simulink model "Ld_Lq_realised_inverter_sinPWM"  (R2021b)
settings: Solver=ode23tb  StartTime=0.0  StopTime=0.16  MaxStep=5e-6  RelTol=1e-3  EnableMultiTasking=on
libraries: spsSeriesRLCBranchLib x18, spsCurrentMeasurementLib x8, spsVoltageMeasurementLib x8, spsMosfetLib x6, simulink x3, spsIdealSwitchLib x1, slpidlib x1, spsThreePhaseSourceLib x1, spspowerguiLib x1
settings Model: SimulationMode=accelerator  Creator=Алексей  LastModifiedBy=alexey
settings SolverCC: ZeroCrossControl=DisableAll  ZeroCrossAlgorithm=Adaptive  AlgebraicLoopSolver=TrustRegion
settings DataIOCC: SaveFormat=Array  SaveOutput=off  SignalLogging=off  DSMLogging=off  SaveTime=off  ReturnWorkspaceOutputs=off
settings OptimizationCC: LifeSpan=inf
settings DebuggingCC: UnderspecifiedInitializationDetection=Classic  MergeDetectMultiDrivingBlocksExec=none  SolverPrmCheckMsg=warning  AllowSymbolicDim=off  SFUnexpectedBacktrackingDiag=warning  SFNoUnconditionalDefaultTransitionDiag=warning  SFExecutionAtInitializationDiag=none  SFMachineParentedDataDiag=warning  ArithmeticOperatorsInVariantConditions=warning
settings HardwareCC: ProdBitPerPointer=32  ProdBitPerSizeT=32  ProdBitPerPtrDiffT=32  ProdLargestAtomicFloat=None  ProdIntDivRoundTo=Undefined  ProdEndianess=Unspecified  ProdWordSize=32  ProdHWDeviceType=32-bit Generic
settings ModelReferenceCC: PropagateSignalLabelsOutOfModel=off
settings SFSimCC: SimUseLocalCustomCode=off  CustomCodeUndefinedFunction=UseInterfaceOnly
settings RTWCC: RTWUseLocalCustomCode=off
settings CodeAppCC: StateflowObjectComments=on
settings GRTTargetCC: TargetLangStandard=C89/C90 (ANSI)  RTWCAPISignals=on  RTWCAPIParams=on
settings ConfigComp: CovMetricSettings=dw  CovSaveCumulativeToWorkspaceVar=on  CovSaveSingleToWorkspaceVar=on  CovExternalEMLEnable=off  CovSFcnEnable=off
settings SimscapeCC: SimscapeNormalizeSystem=off

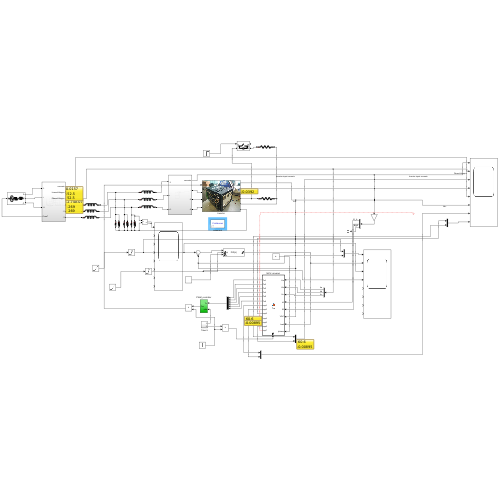
[thumbnail: Simulink's stored preview of the top-level diagram]
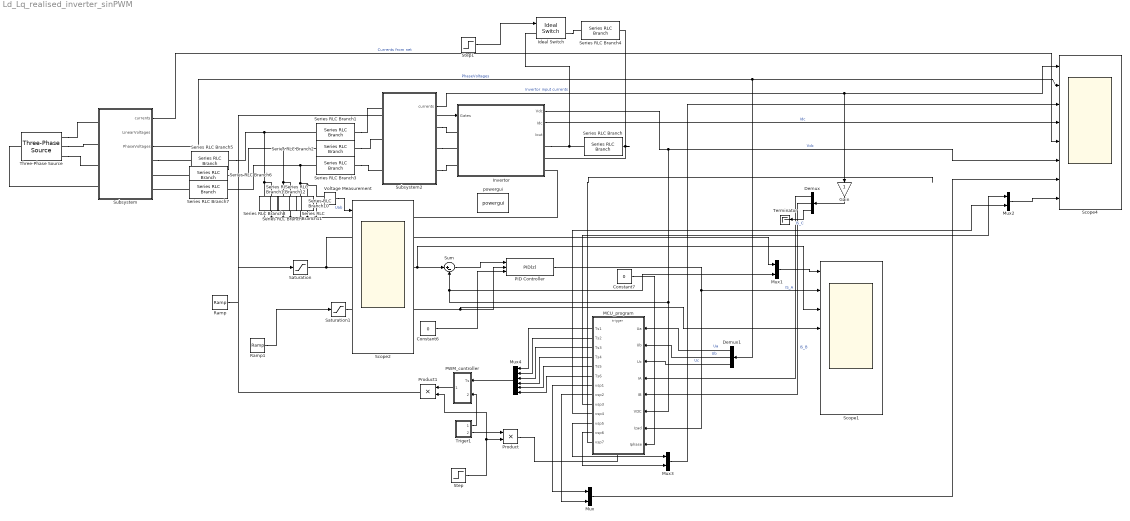
== system Ld_Lq_realised_inverter_sinPWM ==
  Constant6 : Constant  Value=0
  Constant7 : Constant  Value=0
  Demux : Demux  Outputs=3
  Demux1 : Demux  Outputs=3
  Gain : Gain
  Ideal Switch : spsIdealSwitchLib/Ideal Switch  Ron=0.001  Lon=0  IC=0  Rs=1e5  Cs=inf  Measurements=on
  Invertor : Subsystem
      mask Display: image('$imagefile'); % Use "Edit Image" on toolstrip to change.
  MCU_program : MATLAB Function  TreatAsAtomicUnit=on
  Mux{,1..3} (4 alike) : Mux  Inputs=2
  Mux4 : Mux  Inputs=6
  PID Controller : slpidlib/PID Controller  Controller=PID  Form=Parallel  TimeDomain=Discrete-time  UseExternalTs=off  SampleTime=50e-6  IntegratorMethod=Forward Euler  FilterMethod=Forward Euler  ControllerParametersSource=internal  P=3  I=15  D=0  UseFilter=on  N=100  TunerSelectOption=Transfer Function Based (PID Tuner App)  InitialConditionSource=internal  InitialConditionForIntegrator=0  InitialConditionForFilter=0  DifferentiatorICPrevScaledInput=0  ExternalReset=none  TrackingMode=off  Kt=1  LimitOutput=on  SatLimitsSource=external  UpperSaturationLimit=150  LowerSaturationLimit=0  LinearizeAsGain=on  AntiWindupMode=clamping  Kb=1  POutMin=[]  POutMax=[]  IOutMin=[]  IOutMax=[]  DOutMin=[]  DOutMax=[]  NOutMin=[]  NOutMax=[]  SumOutMin=[]  SumOutMax=[]  SaturationOutMin=[]  SaturationOutMax=[]  PParamMin=[]  PParamMax=[]  IParamMin=[]  IParamMax=[]  DParamMin=[]  DParamMax=[]  NParamMin=[]  NParamMax=[]  KbParamMin=[]  KbParamMax=[]  KtParamMin=[]  KtParamMax=[]  KbOutMin=[]  KbOutMax=[]  KtOutMin=[]  KtOutMax=[]  IntegratorOutMin=[]  IntegratorOutMax=[]  FilterOutMin=[]  FilterOutMax=[]  SumI1OutMin=[]  SumI1OutMax=[]  SumI2OutMin=[]  SumI2OutMax=[]  SumI3OutMin=[]  SumI3OutMax=[]  SumI4OutMin=[]  SumI4OutMax=[]  SumDOutMin=[]  SumDOutMax=[]  DifferentiatorOutMin=[]  DifferentiatorOutMax=[]  FilterDiffOutCoefMin=[]  FilterDiffOutCoefMax=[]  ReciprocalOutMin=[]  ReciprocalOutMax=[]  SumDenOutMin=[]  SumDenOutMax=[]  SumNumOutMin=[]  SumNumOutMax=[]  DivideOutMin=[]  DivideOutMax=[]  UdiffTsProdOutMin=[]  UdiffTsProdOutMax=[]  NTsProdOutMin=[]  NTsProdOutMax=[]  UintegralTsProdOutMin=[]  UintegralTsProdOutMax=[]  UngainTsProdOutMin=[]  UngainTsProdOutMax=[]  IntegratorContinuousStateAttributes=''  IntegratorStateMustResolveToSignalObject=off  IntegratorRTWStateStorageClass=Auto  FilterContinuousStateAttributes=''  FilterStateMustResolveToSignalObject=off  FilterRTWStateStorageClass=Auto  ParallelPVariant=InternalParameters  IdealPVariant=Disabled  IVariant=InternalParameters  DVariant=InternalParameters  IntegratorVariant=Discrete  SatVariant=External  AWVariant=DiscClampingParallel  PCopyVariant=Disabled  TRVariant=Disabled  FdbkBlocksVariant=Forward  IdealPFdbkVariant=Disabled  SatFdbkVariant=Disabled  DerivativeFilterVariant=ForwardEulerFilter  NVariant=InternalParameters  NCopyVariant=Disabled  FilterICVariant=InternalICsFilter  IntegratorICVariant=InternalICs  ExternalResetVariant=Disabled  TRSumVariant=Passthrough  SumFdbkVariant=Disabled  SumVariant=Sum_PID  TsampFilterVariant=InternalTs  TsampNgainVariant=Passthrough  TsampIntegralVariant=Passthrough  ExternalSaturationOutDataTypeStr=Inherit: Same as second input
  PWM_controller : Subsystem
  Product : Product
  Product1 : Product
  Ramp : simulink/Sources/Ramp  slope=6500  start=0  InitialOutput=550
  Ramp1 : simulink/Sources/Ramp  slope=15000  start=0  InitialOutput=0
  Saturation : Saturate  UpperLimit=650  LowerLimit=560
  Saturation1 : Saturate  UpperLimit=150  LowerLimit=50
  Scope1 : Scope  NumInputPorts=8
  Scope2 : Scope  NumInputPorts=8
  Scope4 : Scope  NumInputPorts=8
  Series RLC Branch : spsSeriesRLCBranchLib/Series RLC Branch  LConnTagsString=__new0  RConnTagsString=__new0  BranchType=R  Resistance=50  Inductance=1e-3  SetiL0=off  InitialCurrent=0  Capacitance=1e-6  Setx0=off  InitialVoltage=0  Measurements=None
  Series RLC Branch1 : spsSeriesRLCBranchLib/Series RLC Branch  LConnTagsString=__new0  RConnTagsString=__new0  BranchType=L  Resistance=10  Inductance=500e-6  SetiL0=off  InitialCurrent=0  Capacitance=1e-6  Setx0=off  InitialVoltage=0  Measurements=None
  Series RLC Branch10 : spsSeriesRLCBranchLib/Series RLC Branch  LConnTagsString=__new0  RConnTagsString=__new0  BranchType=C  Resistance=10  Inductance=750e-6  SetiL0=off  InitialCurrent=0  Capacitance=1e-12  Setx0=off  InitialVoltage=0  Measurements=None
  Series RLC Branch11 : spsSeriesRLCBranchLib/Series RLC Branch  LConnTagsString=__new0  RConnTagsString=__new0  BranchType=R  Resistance=1e6  Inductance=750e-6  SetiL0=off  InitialCurrent=0  Capacitance=2e-18  Setx0=off  InitialVoltage=0  Measurements=None
  Series RLC Branch12 : spsSeriesRLCBranchLib/Series RLC Branch  LConnTagsString=__new0  RConnTagsString=__new0  BranchType=R  Resistance=1e6  Inductance=750e-6  SetiL0=off  InitialCurrent=0  Capacitance=2e-18  Setx0=off  InitialVoltage=0  Measurements=None
  Series RLC Branch13 : spsSeriesRLCBranchLib/Series RLC Branch  LConnTagsString=__new0  RConnTagsString=__new0  BranchType=R  Resistance=1e6  Inductance=750e-6  SetiL0=off  InitialCurrent=0  Capacitance=2e-18  Setx0=off  InitialVoltage=0  Measurements=None
  Series RLC Branch2 : spsSeriesRLCBranchLib/Series RLC Branch  LConnTagsString=__new0  RConnTagsString=__new0  BranchType=L  Resistance=10  Inductance=500e-6  SetiL0=off  InitialCurrent=0  Capacitance=1e-6  Setx0=off  InitialVoltage=0  Measurements=None
  Series RLC Branch3 : spsSeriesRLCBranchLib/Series RLC Branch  LConnTagsString=__new0  RConnTagsString=__new0  BranchType=L  Resistance=10  Inductance=500e-6  SetiL0=off  InitialCurrent=0  Capacitance=1e-6  Setx0=off  InitialVoltage=0  Measurements=None
  Series RLC Branch4 : spsSeriesRLCBranchLib/Series RLC Branch  LConnTagsString=__new0  RConnTagsString=__new0  BranchType=R  Resistance=20  Inductance=1e-3  SetiL0=off  InitialCurrent=0  Capacitance=1e-6  Setx0=off  InitialVoltage=0  Measurements=None
  Series RLC Branch5 : spsSeriesRLCBranchLib/Series RLC Branch  LConnTagsString=__new0  RConnTagsString=__new0  BranchType=L  Resistance=10  Inductance=5e-6  SetiL0=off  InitialCurrent=0  Capacitance=1e-6  Setx0=off  InitialVoltage=0  Measurements=None
  Series RLC Branch6 : spsSeriesRLCBranchLib/Series RLC Branch  LConnTagsString=__new0  RConnTagsString=__new0  BranchType=L  Resistance=10  Inductance=5e-6  SetiL0=off  InitialCurrent=0  Capacitance=1e-6  Setx0=off  InitialVoltage=0  Measurements=None
  Series RLC Branch7 : spsSeriesRLCBranchLib/Series RLC Branch  LConnTagsString=__new0  RConnTagsString=__new0  BranchType=L  Resistance=10  Inductance=5e-6  SetiL0=off  InitialCurrent=0  Capacitance=1e-6  Setx0=off  InitialVoltage=0  Measurements=None
  Series RLC Branch8 : spsSeriesRLCBranchLib/Series RLC Branch  LConnTagsString=__new0  RConnTagsString=__new0  BranchType=C  Resistance=10  Inductance=750e-6  SetiL0=off  InitialCurrent=0  Capacitance=1e-12  Setx0=off  InitialVoltage=0  Measurements=None
  Series RLC Branch9 : spsSeriesRLCBranchLib/Series RLC Branch  LConnTagsString=__new0  RConnTagsString=__new0  BranchType=C  Resistance=10  Inductance=750e-6  SetiL0=off  InitialCurrent=0  Capacitance=1e-12  Setx0=off  InitialVoltage=0  Measurements=None
  Step : Step  Time=0  SampleTime=0
  Step1 : Step  Time=0.1  SampleTime=0
  Subsystem : Subsystem
  Subsystem2 : Subsystem
  Sum : Sum  Inputs=|+-
  Terminator : Terminator
  Three-Phase Source : spsThreePhaseSourceLib/Three-Phase Source  InternalConnection=Yn  VoltagePhases=on  Voltage=200  PhaseAngle=0  Voltage_phases=[220 220 220]  PhaseAngles_phases=[0 -120 +120]  Frequency=50  NonIdealSource=on  SpecifyImpedance=off  Resistance=1e-6  Inductance=30e-9  ShortCircuitLevel=100e6  BaseVoltage=200  XRratio=7  BusType=swing  Pref=10e3  Qref=0  Prefabc=[10e3, 10e3, 10e3]  Qrefabc=[0, 0, 0]  Qmin=-inf  Qmax=inf
  Triger1 : Subsystem
  Voltage Measurement : spsVoltageMeasurementLib/Voltage Measurement  PhasorSimulation=off  OutputType=Complex  PSBequivalent=0
  powergui : spspowerguiLib/powergui  Priority=1  SimulationMode=Continuous  SampleTime=50e-6  frequency=60  Iterations=50  frequencyindice=0  Pbase=100e6  ErrMax=1e-4  UnitsV=kV  UnitsW=MW  buscounter=0  FunctionMessages=off  echomessages=off  EnableUseOfTLC=off  CurrentSourceSwitches=on  DisableSnubberDevices=off  DisableRonSwitches=off  DisableVfSwitches=off  DisplayEquations=off  AutomaticDiscreteSolvers=off  SolverType=Tustin  Interpol=off  ExternalGateDelay=off  methode=off  Ts=0  x0status=blocks  SPID=off  SwTol=0  HookPort=off  NonlinearTolerance=1e-4  nMaxIteration=100  ContinueOnMaxIteration=off  RestoreLinks=warning  ResistiveCurrentMeasurement=off  Frange=[0:2:500]  Ylog=off  Xlog=on  ShowGrid=off  save=off  variable=ZData  structure=SD2  ZoomFFT=on  StartTime=0.7  cycles=10  DisplayStyle=4  fundamental=382  FreqAxis=off  MaxFrequency=50000  frequencyindicesteady=1  RmsSteady=1  display=off
  wires:
  Demux/1 -> MCU_program/4(IA)  "IS_A"
  Demux/2 -> MCU_program/5(IB)  "IS_B"
  MCU_program/8(vsp2) -> Mux/2
  MCU_program/7(vsp1) -> Mux/1
  MCU_program/6(Ts6) -> Mux4/6
  MCU_program/5(Ts5) -> Mux4/5
  MCU_program/4(Ts4) -> Mux4/4
  MCU_program/3(Ts3) -> Mux4/3
  Triger1/1(1) -> PWM_controller/2(pila)
  Product1/1 -> Invertor/1(Gates)
  MCU_program/1(Ts1) -> Mux4/1
  Mux4/1 -> PWM_controller/1(Ts)
  Product/1 -> MCU_program/Trigger
  MCU_program/2(Ts2) -> Mux4/2
  Invertor/1(Vdc) -> Scope4/6, Mux1/2, Sum/2, MCU_program/6(VDC)  "Vdc"
  Invertor/2(Idc) -> Scope4/4  "Idc"
  Demux/3 -> Terminator/1  "IS_C"
  Demux1/1 -> MCU_program/1(Ua)  "Ua"
  Demux1/2 -> MCU_program/2(Ub)  "Ub"
  Demux1/3 -> MCU_program/3(Uc)  "Uc"
  Subsystem2/1(currents) -> Gain/1, Scope4/1  "Invertor input currents"
  Mux/1 -> Scope4/7
  Subsystem/3(PhaseVoltages) -> Demux1/1, Scope4/2  "PhaseVoltages"
  MCU_program/10(vsp4) -> Mux2/2
  PID Controller/1 -> MCU_program/7(Izad), Scope1/2
  Constant7/1 -> MCU_program/8(Iphase)
  Mux2/1 -> Scope4/8
  MCU_program/9(vsp3) -> Mux2/1
  Triger1/2(2) -> Product/1
  Step/1 -> Product1/2, Product/2
  PWM_controller/1(Tss) -> Product1/1
  MCU_program/11(vsp5) -> Mux3/1
  MCU_program/12(vsp6) -> Mux3/2
  Mux3/1 -> Scope4/3
  MCU_program/13(vsp7) -> ?
  Gain/1 -> Demux/1
  Sum/1 -> PID Controller/1
  Ramp/1 -> Saturation/1
  Step1/1 -> Ideal Switch/1
  Saturation/1 -> Mux1/1, Scope1/3, Sum/1
  Ramp1/1 -> Saturation1/1
  Constant6/1 -> PID Controller/3
  Saturation1/1 -> Scope1/4, PID Controller/2
  Mux1/1 -> Scope1/1
  Subsystem/1(currents) -> Scope4/5  "Currents from net"
  Voltage Measurement/1 -> Scope2/1  "Uab"
  connections:
  Invertor/RConn1 -- Ideal Switch/LConn1 -- Series RLC Branch/LConn1
  Series RLC Branch/RConn1 -- Invertor/RConn2 -- Series RLC Branch4/RConn1
  Series RLC Branch5/RConn1 -- Series RLC Branch13/LConn1 -- Series RLC Branch8/LConn1 -- Series RLC Branch1/LConn1
  Three-Phase Source/RConn1 -- Subsystem/LConn1
  Series RLC Branch2/RConn1 -- Subsystem2/LConn2
  Three-Phase Source/RConn2 -- Subsystem/LConn2
  Three-Phase Source/RConn3 -- Subsystem/LConn3
  Series RLC Branch3/RConn1 -- Subsystem2/LConn3
  Series RLC Branch1/RConn1 -- Subsystem2/LConn1
  Series RLC Branch6/LConn1 -- Subsystem/RConn2
  Series RLC Branch7/LConn1 -- Subsystem/RConn3
  Series RLC Branch8/RConn1 -- Series RLC Branch13/RConn1 -- Series RLC Branch12/RConn1 -- Invertor/RConn3 -- Voltage Measurement/LConn2 -- Series RLC Branch11/RConn1 -- Series RLC Branch10/RConn1 -- Series RLC Branch9/RConn1
  Ideal Switch/RConn1 -- Series RLC Branch4/LConn1
  Subsystem/RConn1 -- Series RLC Branch5/LConn1
  Series RLC Branch2/LConn1 -- Series RLC Branch12/LConn1 -- Series RLC Branch9/LConn1 -- Series RLC Branch6/RConn1
  Series RLC Branch3/LConn1 -- Voltage Measurement/LConn1 -- Series RLC Branch11/LConn1 -- Series RLC Branch10/LConn1 -- Series RLC Branch7/RConn1
  Subsystem2/RConn1 -- Invertor/LConn1
  Subsystem2/RConn2 -- Invertor/LConn2
  Subsystem2/RConn3 -- Invertor/LConn3
  Three-Phase Source/LConn1 -- Subsystem/LConn4

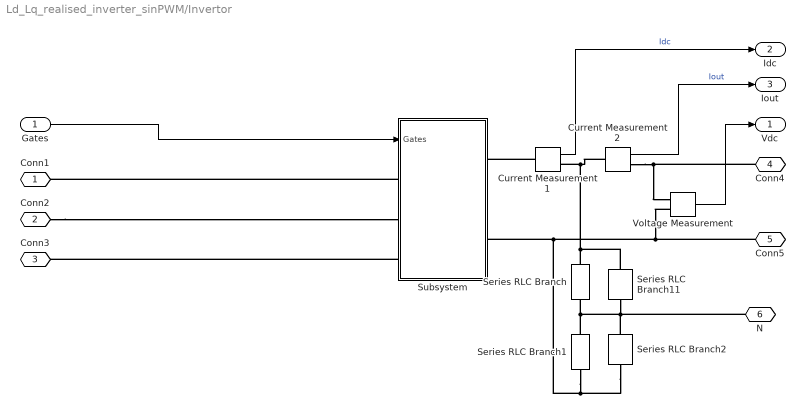
== system Ld_Lq_realised_inverter_sinPWM/Invertor ==
  Gates : Inport
  Current Measurement1 : spsCurrentMeasurementLib/Current Measurement  PhasorSimulation=off  OutputType=Complex  PSBequivalent=0
  Current Measurement2 : spsCurrentMeasurementLib/Current Measurement  PhasorSimulation=off  OutputType=Complex  PSBequivalent=0
  Series RLC Branch : spsSeriesRLCBranchLib/Series RLC Branch  LConnTagsString=__new0  RConnTagsString=__new0  BranchType=C  Resistance=1  Inductance=1e-3  SetiL0=off  InitialCurrent=0  Capacitance=750e-6  Setx0=on  InitialVoltage=270  Measurements=None
  Series RLC Branch1 : spsSeriesRLCBranchLib/Series RLC Branch  LConnTagsString=__new0  RConnTagsString=__new0  BranchType=C  Resistance=1  Inductance=1e-3  SetiL0=off  InitialCurrent=0  Capacitance=750e-6  Setx0=on  InitialVoltage=270  Measurements=None
  Series RLC Branch11 : spsSeriesRLCBranchLib/Series RLC Branch  LConnTagsString=__new0  RConnTagsString=__new0  BranchType=R  Resistance=1e6  Inductance=750e-6  SetiL0=off  InitialCurrent=0  Capacitance=2e-18  Setx0=off  InitialVoltage=0  Measurements=None
  Series RLC Branch2 : spsSeriesRLCBranchLib/Series RLC Branch  LConnTagsString=__new0  RConnTagsString=__new0  BranchType=R  Resistance=1e6  Inductance=750e-6  SetiL0=off  InitialCurrent=0  Capacitance=2e-18  Setx0=off  InitialVoltage=0  Measurements=None
  Subsystem : Subsystem
  Voltage Measurement : spsVoltageMeasurementLib/Voltage Measurement  PhasorSimulation=off  OutputType=Complex  PSBequivalent=0
  Conn1 : PMIOPort  Side=Left
  Conn2 : PMIOPort  Port=2  Side=Left
  Conn3 : PMIOPort  Port=3  Side=Left
  Conn4 : PMIOPort  Port=4  Side=Right
  Conn5 : PMIOPort  Port=5  Side=Right
  N : PMIOPort  Port=6  Side=Right
  Vdc : Outport  VectorParamsAs1DForOutWhenUnconnected=off
  Idc : Outport  Port=2  VectorParamsAs1DForOutWhenUnconnected=off
  Iout : Outport  Port=3  VectorParamsAs1DForOutWhenUnconnected=off
  wires:
  Voltage Measurement/1 -> Vdc/1
  Gates/1 -> Subsystem/1(Gates)
  Current Measurement1/1 -> Idc/1  "Idc"
  Current Measurement2/1 -> Iout/1  "Iout"
  connections:
  Current Measurement1/LConn1 -- Subsystem/RConn1
  Voltage Measurement/LConn2 -- Series RLC Branch2/RConn1 -- Series RLC Branch1/RConn1 -- Subsystem/RConn2 -- Conn5/RConn1
  Subsystem/LConn1 -- Conn1/RConn1
  Conn2/RConn1 -- Subsystem/LConn2
  Subsystem/LConn3 -- Conn3/RConn1
  Conn4/RConn1 -- Current Measurement2/RConn1 -- Voltage Measurement/LConn1
  Current Measurement2/LConn1 -- Series RLC Branch11/LConn1 -- Series RLC Branch/LConn1 -- Current Measurement1/RConn1
  Series RLC Branch1/LConn1 -- N/RConn1 -- Series RLC Branch2/LConn1 -- Series RLC Branch11/RConn1 -- Series RLC Branch/RConn1

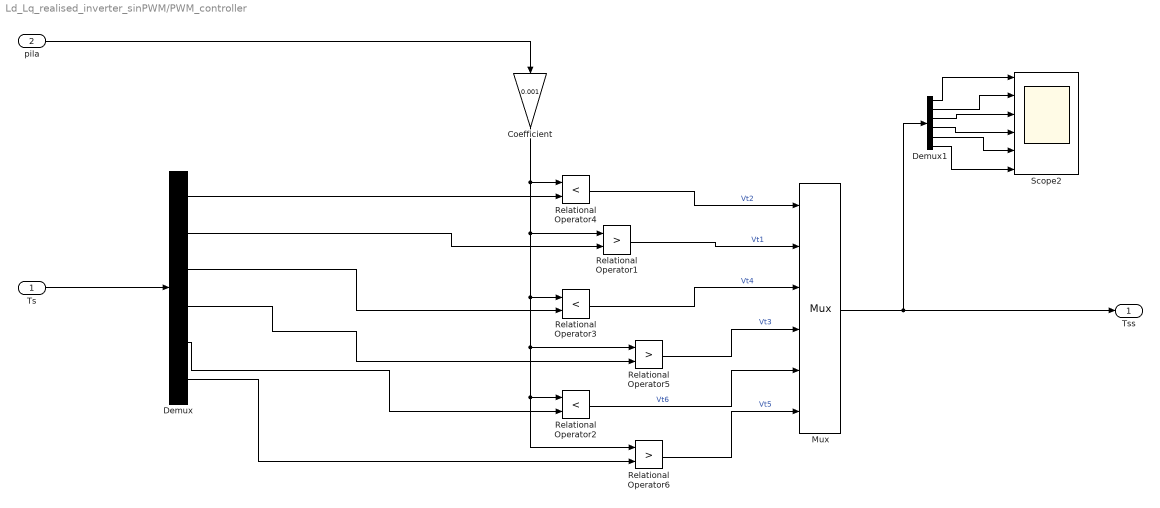
== system Ld_Lq_realised_inverter_sinPWM/PWM_controller ==
  Ts : Inport
  pila : Inport  Port=2
  Coefficient : Gain  Gain=0.001
  Demux : Demux  Outputs=6
  Demux1 : Demux  Outputs=6
  Mux : Mux  Inputs=6
  Relational Operator1 : RelationalOperator  Operator=>  OutDataTypeStr=boolean  RndMeth=Nearest
  Relational Operator2 : RelationalOperator  Operator=<  OutDataTypeStr=boolean  RndMeth=Nearest
  Relational Operator3 : RelationalOperator  Operator=<  OutDataTypeStr=boolean  RndMeth=Nearest
  Relational Operator4 : RelationalOperator  Operator=<  OutDataTypeStr=boolean  RndMeth=Nearest
  Relational Operator5 : RelationalOperator  Operator=>  OutDataTypeStr=boolean  RndMeth=Nearest
  Relational Operator6 : RelationalOperator  Operator=>  OutDataTypeStr=boolean  RndMeth=Nearest
  Scope2 : Scope  NumInputPorts=6
  Tss : Outport  VectorParamsAs1DForOutWhenUnconnected=off
  wires:
  Relational Operator4/1 -> Mux/1  "Vt2"
  Demux/3 -> Relational Operator3/2
  Demux/5 -> Relational Operator2/2
  Relational Operator3/1 -> Mux/3  "Vt4"
  Relational Operator2/1 -> Mux/5  "Vt6"
  Ts/1 -> Demux/1
  Coefficient/1 -> Relational Operator1/1, Relational Operator3/1, Relational Operator5/1, Relational Operator2/1, Relational Operator6/1, Relational Operator4/1
  Relational Operator1/1 -> Mux/2  "Vt1"
  Relational Operator5/1 -> Mux/4  "Vt3"
  Relational Operator6/1 -> Mux/6  "Vt5"
  Demux/2 -> Relational Operator1/2
  Demux/4 -> Relational Operator5/2
  Demux/6 -> Relational Operator6/2
  Demux/1 -> Relational Operator4/2
  pila/1 -> Coefficient/1
  Mux/1 -> Tss/1, Demux1/1
  Demux1/2 -> Scope2/2
  Demux1/1 -> Scope2/1
  Demux1/4 -> Scope2/4
  Demux1/5 -> Scope2/5
  Demux1/6 -> Scope2/6
  Demux1/3 -> Scope2/3

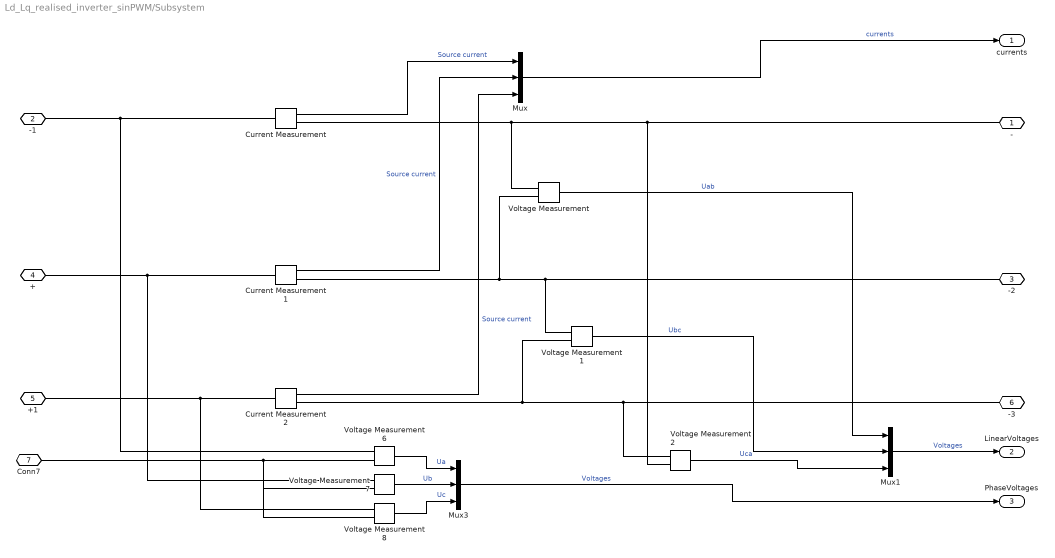
== system Ld_Lq_realised_inverter_sinPWM/Subsystem ==
  Current Measurement : spsCurrentMeasurementLib/Current Measurement  PhasorSimulation=off  OutputType=Complex  PSBequivalent=0
  Current Measurement1 : spsCurrentMeasurementLib/Current Measurement  PhasorSimulation=off  OutputType=Complex  PSBequivalent=0
  Current Measurement2 : spsCurrentMeasurementLib/Current Measurement  PhasorSimulation=off  OutputType=Complex  PSBequivalent=0
  Mux : Mux  Inputs=3
  Mux1 : Mux  Inputs=3
  Mux3 : Mux  Inputs=3
  Voltage Measurement{,1..2,6..8} (6 alike) : spsVoltageMeasurementLib/Voltage Measurement  PhasorSimulation=off  OutputType=Complex  PSBequivalent=0
  - : PMIOPort  Side=Right
  -1 : PMIOPort  Port=2  Side=Left
  -2 : PMIOPort  Port=3  Side=Right
  + : PMIOPort  Port=4  Side=Left
  +1 : PMIOPort  Port=5  Side=Left
  -3 : PMIOPort  Port=6  Side=Right
  Conn7 : PMIOPort  Port=7  Side=Left
  currents : Outport
  LinearVoltages : Outport  Port=2
  PhaseVoltages : Outport  Port=3
  wires:
  Current Measurement2/1 -> Mux/3  "Source current"
  Current Measurement1/1 -> Mux/2  "Source current"
  Voltage Measurement1/1 -> Mux1/2  "Ubc"
  Voltage Measurement2/1 -> Mux1/3  "Uca"
  Mux/1 -> currents/1  "currents"
  Voltage Measurement/1 -> Mux1/1  "Uab"
  Current Measurement/1 -> Mux/1  "Source current"
  Mux1/1 -> LinearVoltages/1  "Voltages"
  Mux3/1 -> PhaseVoltages/1  "Voltages"
  Voltage Measurement8/1 -> Mux3/3  "Uc"
  Voltage Measurement6/1 -> Mux3/1  "Ua"
  Voltage Measurement7/1 -> Mux3/2  "Ub"
  connections:
  -1/RConn1 -- Voltage Measurement6/LConn1 -- Current Measurement/LConn1
  Current Measurement1/RConn1 -- Voltage Measurement/LConn2 -- -2/RConn1 -- Voltage Measurement1/LConn1
  Current Measurement/RConn1 -- Voltage Measurement/LConn1 -- Voltage Measurement2/LConn2 -- -/RConn1
  Current Measurement2/RConn1 -- Voltage Measurement2/LConn1 -- -3/RConn1 -- Voltage Measurement1/LConn2
  Voltage Measurement6/LConn2 -- Voltage Measurement8/LConn2 -- Voltage Measurement7/LConn2 -- Conn7/RConn1
  +1/RConn1 -- Voltage Measurement8/LConn1 -- Current Measurement2/LConn1
  +/RConn1 -- Voltage Measurement7/LConn1 -- Current Measurement1/LConn1

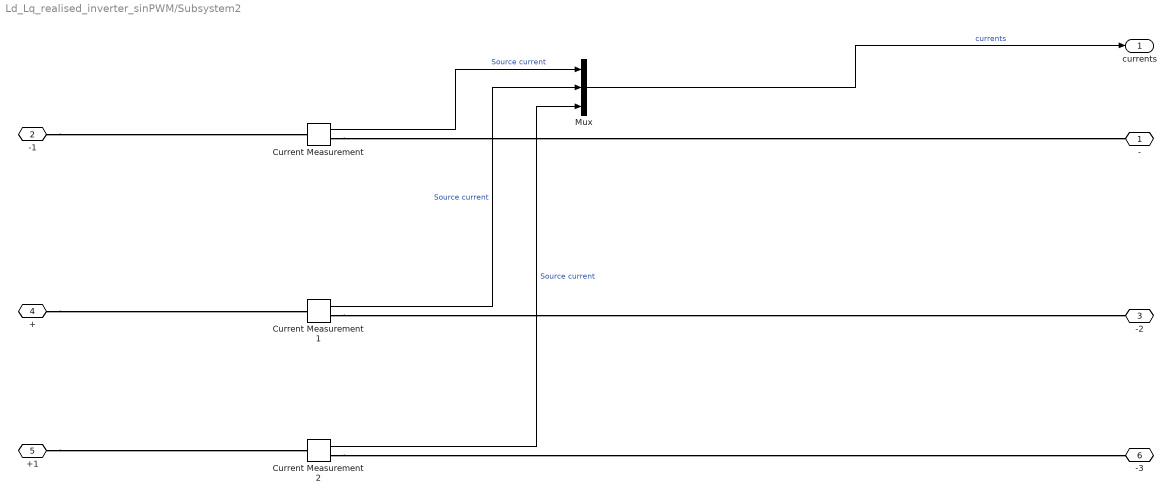
== system Ld_Lq_realised_inverter_sinPWM/Subsystem2 ==
  Current Measurement : spsCurrentMeasurementLib/Current Measurement  PhasorSimulation=off  OutputType=Complex  PSBequivalent=0
  Current Measurement1 : spsCurrentMeasurementLib/Current Measurement  PhasorSimulation=off  OutputType=Complex  PSBequivalent=0
  Current Measurement2 : spsCurrentMeasurementLib/Current Measurement  PhasorSimulation=off  OutputType=Complex  PSBequivalent=0
  Mux : Mux  Inputs=3
  - : PMIOPort  Side=Right
  -1 : PMIOPort  Port=2  Side=Left
  -2 : PMIOPort  Port=3  Side=Right
  + : PMIOPort  Port=4  Side=Left
  +1 : PMIOPort  Port=5  Side=Left
  -3 : PMIOPort  Port=6  Side=Right
  currents : Outport
  wires:
  Current Measurement/1 -> Mux/1  "Source current"
  Mux/1 -> currents/1  "currents"
  Current Measurement1/1 -> Mux/2  "Source current"
  Current Measurement2/1 -> Mux/3  "Source current"
  connections:
  +/RConn1 -- Current Measurement1/LConn1
  +1/RConn1 -- Current Measurement2/LConn1
  Current Measurement2/RConn1 -- -3/RConn1
  Current Measurement/RConn1 -- -/RConn1
  Current Measurement1/RConn1 -- -2/RConn1
  -1/RConn1 -- Current Measurement/LConn1

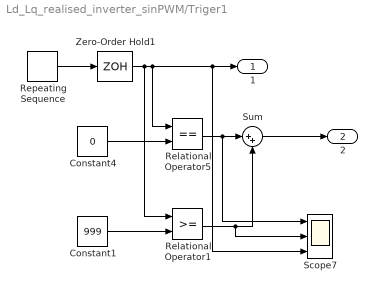
== system Ld_Lq_realised_inverter_sinPWM/Triger1 ==
  Constant1 : Constant  Value=999
  Constant4 : Constant  Value=0
  Relational Operator1 : RelationalOperator  OutDataTypeStr=boolean  RndMeth=Nearest
  Relational Operator5 : RelationalOperator  Operator===  OutDataTypeStr=boolean  RndMeth=Nearest
  Repeating Sequence : simulink/Sources/Repeating Sequence  rep_seq_t=[0 10e-6 20e-6]  rep_seq_y=[0 1000 0]
  Scope7 : Scope  NumInputPorts=3
  Sum : Sum  Inputs=|++
  Zero-Order Hold1 : ZeroOrderHold  SampleTime=5e-8
  1 : Outport  VectorParamsAs1DForOutWhenUnconnected=off
  2 : Outport  Port=2  VectorParamsAs1DForOutWhenUnconnected=off
  wires:
  Zero-Order Hold1/1 -> Relational Operator1/1, Relational Operator5/1, Scope7/3, 1/1
  Repeating Sequence/1 -> Zero-Order Hold1/1
  Constant4/1 -> Relational Operator5/2
  Sum/1 -> 2/1
  Constant1/1 -> Relational Operator1/2
  Relational Operator5/1 -> Scope7/1, Sum/1
  Relational Operator1/1 -> Scope7/2, Sum/2

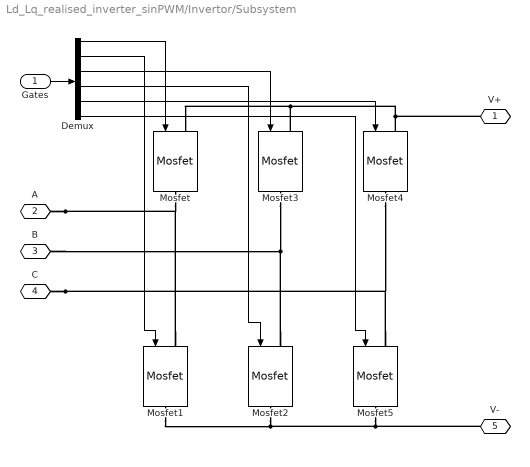
== system Ld_Lq_realised_inverter_sinPWM/Invertor/Subsystem ==
  Gates : Inport
  Demux : Demux  Outputs=6
  Mosfet{,1..5} (6 alike) : spsMosfetLib/Mosfet  Ron=2e-3  Lon=0  Rd=0.01  Vfd=4  IC=0  Rs=1e5  Cs=inf  Measurements=off
  V+ : PMIOPort  Side=Right
  A : PMIOPort  Port=2  Side=Left
  B : PMIOPort  Port=3  Side=Left
  C : PMIOPort  Port=4  Side=Left
  V- : PMIOPort  Port=5  Side=Right
  wires:
  Demux/4 -> Mosfet2/1
  Demux/2 -> Mosfet1/1
  Demux/5 -> Mosfet4/1
  Demux/3 -> Mosfet3/1
  Demux/6 -> Mosfet5/1
  Demux/1 -> Mosfet/1
  Gates/1 -> Demux/1
  connections:
  C/RConn1 -- Mosfet5/LConn1 -- Mosfet4/RConn1
  V-/RConn1 -- Mosfet5/RConn1 -- Mosfet2/RConn1 -- Mosfet1/RConn1
  B/RConn1 -- Mosfet2/LConn1 -- Mosfet3/RConn1
  V+/RConn1 -- Mosfet3/LConn1 -- Mosfet/LConn1 -- Mosfet4/LConn1
  A/RConn1 -- Mosfet/RConn1 -- Mosfet1/LConn1

== matlab function Ld_Lq_realised_inverter_sinPWM/MCU_program ==
  data: Ua input; Ub input; Uc input; IA input; IB input; Ts1 output; Ts2 output; Ts3 output; Ts4 output; Ts5 output; Ts6 output; vsp1 output; vsp2 output; vsp3 output; vsp4 output; VDC input; Izad input; Iphase input; vsp5 output; vsp6 output; vsp7 output
  events: trigger input RISING_EDGE_EVENT
function [Ts1,Ts2,Ts3,Ts4,Ts5,Ts6,vsp1,vsp2,vsp3,vsp4,vsp5,vsp6,vsp7] = fcn(Ua,Ub,Uc,IA,IB,VDC, Izad, Iphase)
%время 1/2 ШИМ периода
dt = 10e-6;

dead_time = 0.0;

kuqp = 8;
kuqi = 5000;

kudp = 5;
kudi = 5000;


persistent Uqint;
if isempty(Uqint)
    Uqint=0;
end 
persistent Udint;
if isempty(Udint)
    Udint=0;
end 


%Преобразования Кларка
Ialfa = -IA;
Ibeta = -(2*IB+IA)/sqrt(3);


Ualfa = Ua;
Ubeta = (2*Ub+Ua)/sqrt(3);

U_ampl = sqrt(Ualfa^2+Ubeta^2);
teta=acos(Ualfa/U_ampl)*sign(Ubeta)+(sign(Ubeta)-1)*(-pi);



%реальные значения токов Id и Iq, полученные через  угол и оси альфа,бета 
Iact = Ialfa*cos(teta)+Ibeta*sin(teta);
Iact = -Iact; %Перевод в систему координат инвертора - для него поглащается активный ток сети
Ireact = Ibeta*cos(teta)-Ialfa*sin(teta); 

Ireact_zad = -Izad * sin(Iphase);

%ПИ-регулятор для напряжения по оси Ку
direact = Ireact_zad - Ireact;
Uqpr = direact * kuqp;
Uqint=Uqint+direact*kuqi*dt;


Iact_zad = Izad * cos(Iphase);
%ПИ-регулятор для напряжения по оси Дэ
diact = Iact_zad - Iact;
Udpr = diact*kudp;
Udint = Udint + diact * kudi * dt;

Um = (2/3)*VDC/sqrt(Uqpr^2+Udpr^2)*0.85;

if(Um<1)
  Uqpr = Uqpr * Um;
  Udpr = Udpr * Um;
end

  
U_q=Uqpr+Uqint;                    
U_d=Udpr+Udint;


%U_q = 0;
U_d = -U_d;



Ua0=U_d*cos(teta)-U_q*sin(teta);
Ub0=U_d*sin(teta)+U_q*cos(teta);



vrefa=sqrt(Ua0^2+Ub0^2);
tetaV = acos(Ua0/vrefa)*sign(Ub0)+(sign(Ub0)-1)*(-pi);

vsp1=Ualfa;
vsp2=Ua0;
vsp3=Ubeta;
vsp4=Ub0;
vsp5 = Iact;
vsp6 = Ireact;
vsp7 = teta;



%алгоритм формирования векторной ШИМ  мертвым веменем dead [мкс]

dead_time=dead_time/(dt*1e6);
a=tetaV;
v2=vrefa*1.5;
if a>=0 && a<pi/3 
    n=1;
elseif  a>=pi/3 && a<2*pi/3 
    n=2;
elseif  a>=2*pi/3 && a<pi 
    n=3;
elseif  a>=pi && a<4*pi/3 
    n=4;
elseif  a>=4*pi/3 && a<5*pi/3 
    n=5;
else n=6;

end

a_cor=a-(n-1)*pi/3;

T1 = (v2/VDC)*sin(pi/3-a_cor)/sin(pi/3);
T2 = (v2/VDC)*sin(a_cor)/sin(pi/3);
T0 = 1 - T1 - T2;
Ta1=0; Ta3=0; Ta5=0; 
switch n
    case 1
        
        Ta1=T1+T2+T0/2;
        
        Ta3=T2+T0/2;
       
        Ta5=T0/2;
       
    case 2
        
        Ta1=T1+T0/2;
        
        Ta3=T1+T2+T0/2;
    
        Ta5=T0/2;       
        
    case 3
        
        Ta1=T0/2;
       
        Ta3=T1+T2+T0/2;
       
        Ta5=T2+T0/2;    
        
    case 4
        
        Ta1=T0/2;
       
        Ta3=T1+T0/2;
       
        Ta5=T1+T2+T0/2;   
       
    case 5
        
        Ta1=T2+T0/2;
        
        Ta3=T0/2;
        
        Ta5=T1+T2+T0/2;     
        
    case 6
        
        Ta1=T1+T2+T0/2;
        
        Ta3=T0/2;
     
        Ta5=T1+T0/2;    
        
end;


Ts1=(Ta1)-dead_time/2; 
Ts3=(Ta3)-dead_time/2; 
Ts5=(Ta5)-dead_time/2;
Ts2=(Ta1)+dead_time/2; 
Ts4=(Ta3)+dead_time/2; 
Ts6=(Ta5)+dead_time/2;


if (IA>0) 
    Ts1=Ts1-dead_time/2;
    Ts2=Ts2-dead_time/2;
else
    Ts1=Ts1+dead_time/2;
    Ts2=Ts2+dead_time/2;           
end;
if (IB>0) 
    Ts3=Ts3-dead_time/2;
    Ts4=Ts4-dead_time/2;
else
    Ts3=Ts3+dead_time/2;
    Ts4=Ts4+dead_time/2; 
end;  
if ((-IA-IB)>0) 
    Ts5=Ts5-dead_time/2;
    Ts6=Ts6-dead_time/2;
else
    Ts5=Ts5+dead_time/2;
    Ts6=Ts6+dead_time/2;           
end;



 






return;
